simulink model "untitled"  (Simulink 7.5)
settings: Solver=ode45  StartTime=0.0  StopTime=200  RelTol=1e-3
settings Model: Creator=Fer  LastModifiedBy=Fer

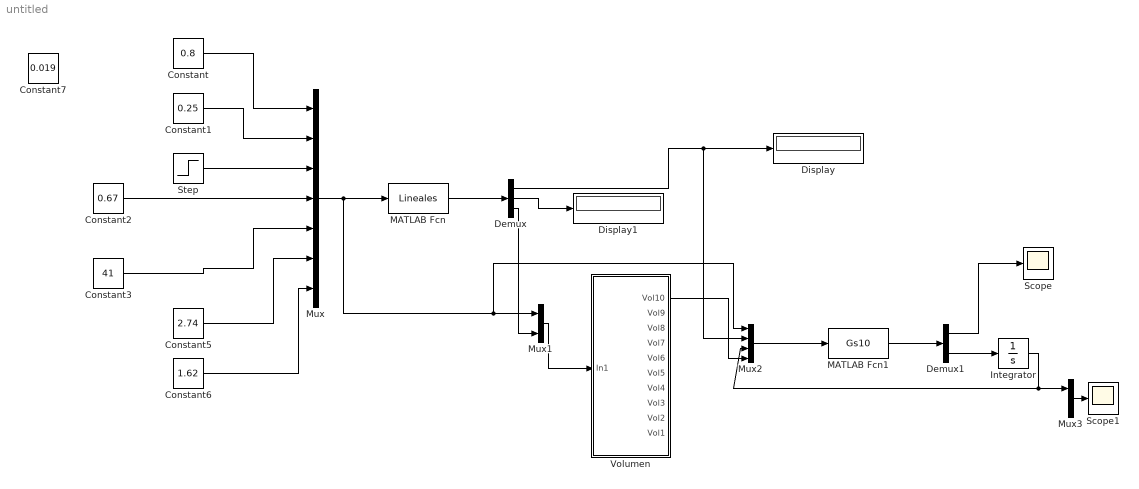
== system untitled ==
  Constant : Constant  Value=0.8  OutDataType=fixdt(1, 16)  OutScaling=2^0
  Constant1 : Constant  Value=0.25  OutDataType=fixdt(1, 16)  OutScaling=2^0
  Constant2 : Constant  Value=0.67  OutDataType=fixdt(1, 16)  OutScaling=2^0
  Constant3 : Constant  Value=41  OutDataType=fixdt(1, 16)  OutScaling=2^0
  Constant5 : Constant  Value=2.74  OutDataType=fixdt(1, 16)  OutScaling=2^0
  Constant6 : Constant  Value=1.62  OutDataType=fixdt(1, 16)  OutScaling=2^0
  Constant7 : Constant  Value=0.019  OutDataType=fixdt(1, 16)  OutScaling=2^0
  Demux : Demux  Outputs=3
  Demux1 : Demux  Outputs=2
  Display : Display
  Display1 : Display
  Integrator : Integrator  InitialCondition=1.6
  MATLAB Fcn : MATLABFcn  MATLABFcn=Lineales
  MATLAB Fcn1 : MATLABFcn  MATLABFcn=Gs10
  Mux : Mux  Inputs=7
  Mux1 : Mux  Inputs=2
  Mux2 : Mux
  Mux3 : Mux  Inputs=2
  Scope : Scope
  Scope1 : Scope
      settings: TimeRange=2.5  YMin=0  YMax=2
  Step : Step  Time=50  Before=0.019  After=0.23  SampleTime=0
  Volumen : Subsystem
  wires:
  Constant/1 -> Mux/1
  Constant1/1 -> Mux/2
  Step/1 -> Mux/3
  Constant3/1 -> Mux/5
  Constant5/1 -> Mux/6
  Constant6/1 -> Mux/7
  Mux/1 -> MATLAB Fcn/1, Mux1/1, Mux2/1
  MATLAB Fcn/1 -> Demux/1
  Demux/1 -> Display/1, Mux2/2
  Mux1/1 -> Volumen/1(In1)
  Mux2/1 -> MATLAB Fcn1/1
  MATLAB Fcn1/1 -> Demux1/1
  Demux1/2 -> Integrator/1
  Integrator/1 -> Mux3/1, Mux2/3
  Demux1/1 -> Scope/1
  Volumen/1(Vol10) -> Mux2/4
  Mux3/1 -> Scope1/1
  Demux/3 -> Mux1/2
  Constant2/1 -> Mux/4
  Demux/2 -> Display1/1

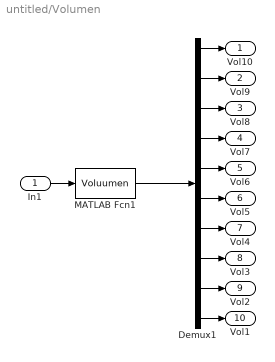
== system untitled/Volumen ==
  In1 : Inport
  Demux1 : Demux  Outputs=10
  MATLAB Fcn1 : MATLABFcn  MATLABFcn=Voluumen
  Vol10 : Outport
  Vol9 : Outport  Port=2
  Vol8 : Outport  Port=3
  Vol7 : Outport  Port=4
  Vol6 : Outport  Port=5
  Vol5 : Outport  Port=6
  Vol4 : Outport  Port=7
  Vol3 : Outport  Port=8
  Vol2 : Outport  Port=9
  Vol1 : Outport  Port=10
  wires:
  MATLAB Fcn1/1 -> Demux1/1
  Demux1/1 -> Vol10/1
  Demux1/2 -> Vol9/1
  Demux1/3 -> Vol8/1
  Demux1/4 -> Vol7/1
  Demux1/5 -> Vol6/1
  In1/1 -> MATLAB Fcn1/1
  Demux1/6 -> Vol5/1
  Demux1/7 -> Vol4/1
  Demux1/8 -> Vol3/1
  Demux1/9 -> Vol2/1
  Demux1/10 -> Vol1/1
